simulink model "Hyduallic_reservoir_simulink"  (R2024b)
settings: Solver=VariableStepAuto  StartTime=0.0  StopTime=10  RelTol=1e-3
libraries: simulink x1
settings Model: PacingRate=0.700000  Creator=theta  LastModifiedBy=theta

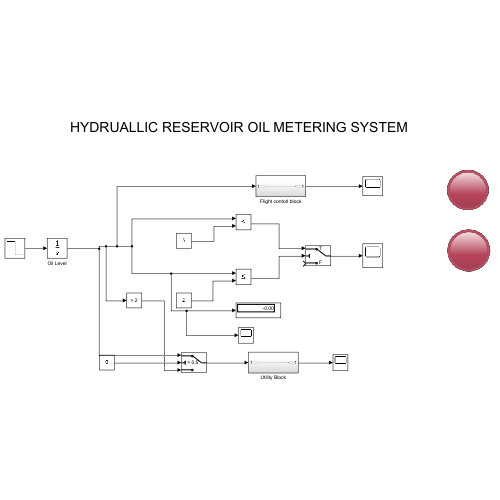
[thumbnail: Simulink's stored preview of the top-level diagram]
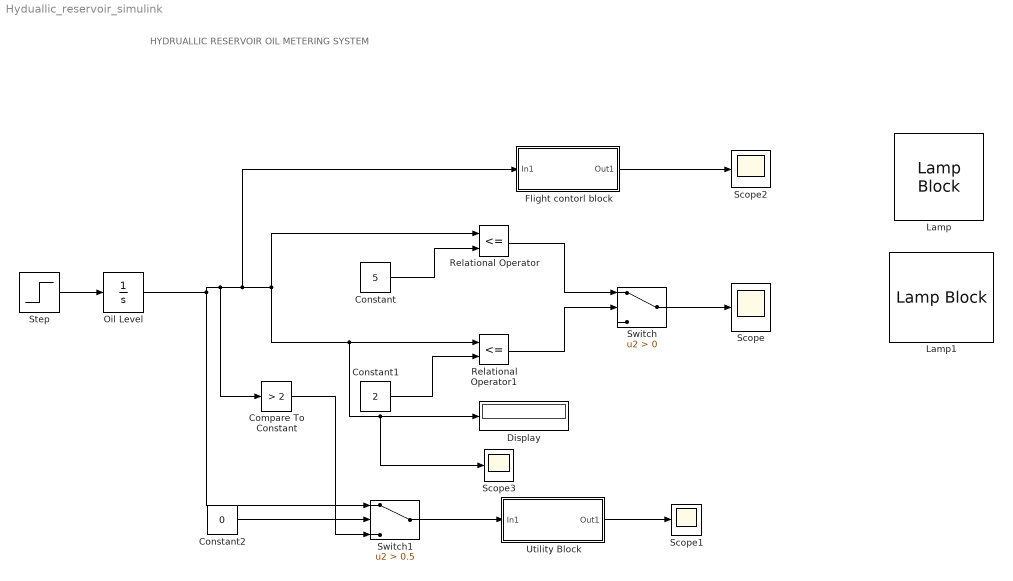
== system Hyduallic_reservoir_simulink ==
  note: HYDRUALLIC RESERVOIR OIL METERING SYSTEM
  Compare To Constant : simulink/Logic and Bit Operations/Compare To Constant  relop=>  const=2  OutDataTypeStr=boolean
  Constant : Constant  Value=5
  Constant1 : Constant  Value=2
  Constant2 : Constant  Value=0
  Display : Display
      settings: Format=bank
  Flight contorl block : Subsystem
  Lamp : LampBlock  LabelPosition=Hide
  Lamp1 : LampBlock  LabelPosition=Hide
  Oil Level : Integrator  InitialCondition=10
  Relational Operator : RelationalOperator  Operator=<=  OutDataTypeStr=boolean  RndMeth=Simplest  InputSameDT=off
  Relational Operator1 : RelationalOperator  Operator=<=  OutDataTypeStr=boolean  RndMeth=Simplest  InputSameDT=off
  Scope{,1..3} (4 alike) : Scope
  Step : Step  Time=0  After=-1  SampleTime=0
  Switch : Switch  Criteria=u2 > Threshold  SaturateOnIntegerOverflow=off  InputSameDT=off
  Switch1 : Switch  Criteria=u2 > Threshold  Threshold=0.5  SaturateOnIntegerOverflow=off  InputSameDT=off
  Utility Block : Subsystem
  wires:
  Step/1 -> Oil Level/1
  Constant1/1 -> Relational Operator1/2
  Constant/1 -> Relational Operator/2
  Oil Level/1 -> Flight contorl block/1(In1), Scope3/1, Display/1, Relational Operator1/1, Relational Operator/1, Compare To Constant/1, Switch1/1
  Relational Operator/1 -> Switch/1
  Relational Operator1/1 -> Switch/2
  Switch/1 -> Scope/1
  Switch1/1 -> Utility Block/1(In1)
  Utility Block/1(Out1) -> Scope1/1
  Flight contorl block/1(Out1) -> Scope2/1
  Compare To Constant/1 -> Switch1/3
  Constant2/1 -> Switch1/2

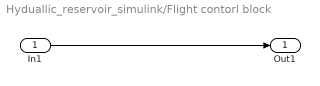
== system Hyduallic_reservoir_simulink/Flight contorl block ==
  In1 : Inport
  Out1 : Outport
  wires:
  In1/1 -> Out1/1

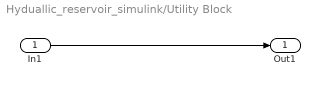
== system Hyduallic_reservoir_simulink/Utility Block ==
  In1 : Inport
  Out1 : Outport
  wires:
  In1/1 -> Out1/1
